simulink model "ClosedLoopSystem_PID"  (R2021a)
settings: Solver=VariableStepAuto  StartTime=0.0  StopTime=10  RelTol=1e-3  AbsTol=1e-3
undefined symbols (not defined in the file or in its folder): dphi0, dtheta0, phi0, ref_angle, theta0
libraries: checkpacklib x2, angle_lib x2, pendulumLib x1
settings Model: DataDictionary=sys_PID_data.sldd  Creator=tshintai  LastModifiedBy=tshintai
settings SolverCC: AutoScaleAbsTol=off
settings ExplorerConfigSet: InternalSimMechanicsExplorerSettings="<ExplorerConfiguration><canonicalview>default</canonicalview><AnimationSetting><BasePlaybackSpeed>1.0</BasePlaybackSpeed><PlaybackSpeedFactor>1.0</PlaybackSpeedFactor></AnimationSetting><TilePanel><TileInfo><Tiles Columns=\"1\" Count=\"1\" Rows=\"1\"><Column Weight=\"1\"/><Row Weight=\"1\"/><Tile Height=\"1\" Width=\"1\" X=\"0\" Y=\"0\"/></Tiles></TileInfo><SceneInfo><SceneViewer><BGColor><R>0.60000002384185791</R><G>0.60000002384185791</G><B>0.60000002384185791</B></BGColor><Camera><DoPerspective>on</DoPerspective><Position><X>0.288190483110498386</X><Y>0.188909908758343986</Y><Z>0.188907569094504485</Z></Position><Center><X>0.00856951562064056649</X><Y>0.00517700605154777782</Y><Z>0.0520990614381798556</Z></Center><Up><X>-0.300028111123132935</X><Y>-0.232308075042136963</Y><Z>0.92521137628441541</Z></Up><ViewLimDist>1</ViewLimDist><YLim>0.466307658154998583</YLim><XLim>0.671250703643049618</XLim></Camera></SceneViewer></SceneInfo></TilePanel><MechEditorPanel><Cameras><Camera><Id>Camera1</Id><Value><Name>Camera1</Name><NativeCamera><PositionKeyframeSet><Keyframe><Time>0</Time><Value><X>0.28819048311049839</X><Y>0.18890990875834399</Y><Z>0.18890756909450448</Z></Value></Keyframe></PositionKeyframeSet><CenterKeyframeSet><Keyframe><Time>0</Time><Value><X>0.0085695156206405665</X><Y>0.0051770060515477778</Y><Z>0.052099061438179856</Z></Value></Keyframe></CenterKeyframeSet><UpVectorKeyframeSet><Keyframe><Time>0</Time><Value><X>-0.30002811112313293</X><Y>-0.23230807504213696</Y><Z>0.92521137628441541</Z></Value></Keyframe></UpVectorKeyframeSet></NativeCamera></Value></Camera></Cameras><GfxPanelCameraMap><MapElement CameraMLId=\"Camera1\" GfxPanelIndex=\"0\"/></GfxPanelCameraMap><VideoCreator><PlaybackSpeedRatio>1.0</PlaybackSpeedRatio><FrameRate>30</FrameRate><VideoFormat>Motion JPEG AVI</VideoFormat><FrameSize>auto</FrameSize></VideoCreator></MechEditorPanel></ExplorerConfiguration>"

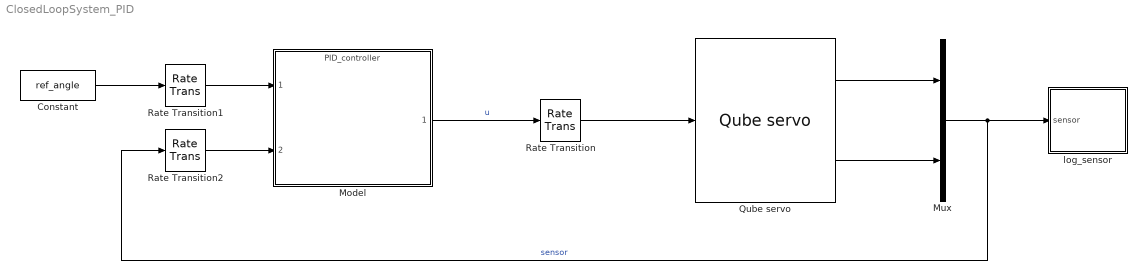
== system ClosedLoopSystem_PID ==
  Constant : Constant  Value=ref_angle
  Model : ModelReference  ModelNameDialog=PID_controller.slx  SimulationMode=Normal  ModelReferenceVersion=1.52
  Mux : Mux  Inputs=2
  Qube servo : pendulumLib/Qube servo  a0=[theta0, phi0]  w0=[dtheta0, dphi0]  R_m=R_m  L_m=L_m  mu_m=mu_m  K_b=K_b_2  n=n  rod_mass=m_r  rod_length=L_r  rod_rad=rod_rad  p_mass=m_p  p_length=L_p  p_rad=p_rad  D_r=D_r_2  D_p=D_p
  Rate Transition : RateTransition
  Rate Transition1 : RateTransition  OutPortSampleTime=ts_PID
  Rate Transition2 : RateTransition  OutPortSampleTime=ts_PID
  log_sensor : Subsystem
  wires:
  Rate Transition/1 -> Qube servo/1
  Qube servo/1 -> Mux/1
  Qube servo/2 -> Mux/2
  Model/1 -> Rate Transition/1  "u"
  Mux/1 -> Rate Transition2/1, log_sensor/1(sensor)  "sensor"
  Constant/1 -> Rate Transition1/1
  Rate Transition1/1 -> Model/1
  Rate Transition2/1 -> Model/2

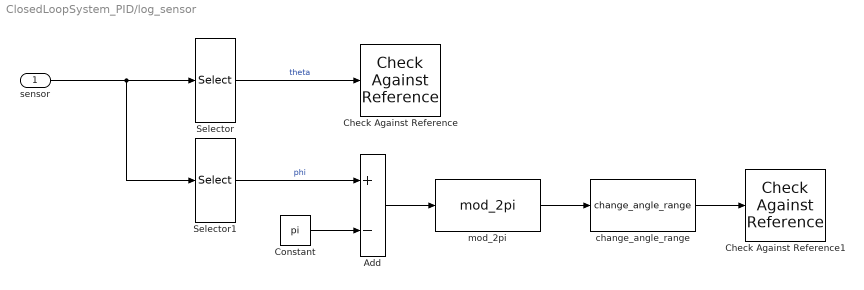
== system ClosedLoopSystem_PID/log_sensor ==
  sensor : Inport
  Add : Sum  Inputs=+-
  Check Against Reference : checkpacklib/Check Against Reference  InstantiateOnLoad=on  enabled=off  stopWhenAssertionFail=off  export=off  ViewDlgPos=[100 200 510 390]  OpenViewOnLoad=off  LaunchViewOnOpen=off  TimeUnits=seconds  EnableReferenceBound=on  AbsTolerance=eps^(1/3)  RelTolerance=0.01  ReferenceTimes=[0, 1]  ReferenceAmplitudes=[0, 0]
      settings: SourceProductBaseCode=CT,ID,MT,SO
  Check Against Reference1 : checkpacklib/Check Against Reference  InstantiateOnLoad=on  enabled=off  stopWhenAssertionFail=off  export=off  ViewDlgPos=[100 200 510 390]  OpenViewOnLoad=off  LaunchViewOnOpen=off  TimeUnits=seconds  EnableReferenceBound=on  AbsTolerance=eps^(1/3)  RelTolerance=0.01  ReferenceTimes=[0, 1]  ReferenceAmplitudes=[0, 0]
      settings: SourceProductBaseCode=CT,ID,MT,SO
  Constant : Constant  Value=pi
  Selector : Selector  InputPortWidth=4  IndexOptions=Index vector (dialog)  Indices=[1]  OutputSizes=1
  Selector1 : Selector  InputPortWidth=4  IndexOptions=Index vector (dialog)  Indices=[2]  OutputSizes=1
  change_angle_range : angle_lib/change_angle_range  SystemSampleTime=-1  VariantActivationTime=update diagram  Latency=0  AutoFrameSizeCalculation=off
  mod_2pi : angle_lib/mod_2pi  SystemSampleTime=-1  VariantActivationTime=update diagram  Latency=0  AutoFrameSizeCalculation=off
  wires:
  sensor/1 -> Selector1/1, Selector/1
  Selector/1 -> Check Against Reference/1  "theta"
  Selector1/1 -> Add/1  "phi"
  Constant/1 -> Add/2
  mod_2pi/1 -> change_angle_range/1
  Add/1 -> mod_2pi/1
  change_angle_range/1 -> Check Against Reference1/1
